simulink model "fim_15_invert"  (R2020b)
settings: Solver=ode4  StartTime=0.0  StopTime=100  RelTol=1e-3  EnableMultiTasking=on
PreLoadFcn:
  | noise_factor=1;
  | load sf_aircraft_buses;
model workspace (MAT data in the model file):
  amp_cmd = 0.119224712533
undefined symbols (not defined in the file): sf_aircraft_ModeType, sigbuilder_block
libraries: simulink x21, sf_aircraft_screen_library x7, simulink_need_slupdate x2
(part 2 of 2)

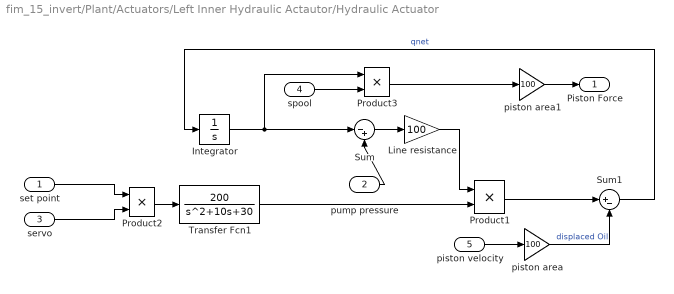
== system fim_15_invert/Plant/Actuators/Left Inner Hydraulic Actautor/Hydraulic Actuator ==
  set point : Inport
  pump pressure : Inport  Port=2
  servo : Inport  Port=3
  spool : Inport  Port=4
  piston velocity : Inport  Port=5
  Integrator : Integrator
  Line resistance : Gain  Gain=100  SaturateOnIntegerOverflow=on  OutDataTypeStr=Inherit: Same as input  ParamDataTypeStr=Inherit: Same as input
  Product1 : Product  SaturateOnIntegerOverflow=on  OutDataTypeStr=Inherit: Same as first input
  Product2 : Product  SaturateOnIntegerOverflow=on  OutDataTypeStr=Inherit: Same as first input
  Product3 : Product  SaturateOnIntegerOverflow=on  OutDataTypeStr=Inherit: Same as first input
  Sum : Sum  Inputs=|-+  SaturateOnIntegerOverflow=on
  Sum1 : Sum  Inputs=|+-  SaturateOnIntegerOverflow=on
  Transfer Fcn1 : TransferFcn  Numerator=[200]  Denominator=[1 10 30]
  piston area : Gain  Gain=100  SaturateOnIntegerOverflow=on  OutDataTypeStr=Inherit: Same as input  ParamDataTypeStr=Inherit: Same as input
  piston area1 : Gain  Gain=100  SaturateOnIntegerOverflow=on  OutDataTypeStr=Inherit: Same as input  ParamDataTypeStr=Inherit: Same as input
  Piston Force : Outport
  wires:
  spool/1 -> Product3/2
  Product3/1 -> piston area1/1
  servo/1 -> Product2/2
  Product2/1 -> Transfer Fcn1/1
  set point/1 -> Product2/1
  piston area1/1 -> Piston Force/1
  pump pressure/1 -> Sum/2
  Integrator/1 -> Sum/1, Product3/1
  Sum1/1 -> Integrator/1  "qnet"
  piston area/1 -> Sum1/2  "displaced Oil"
  piston velocity/1 -> piston area/1
  Product1/1 -> Sum1/1
  Transfer Fcn1/1 -> Product1/2
  Line resistance/1 -> Product1/1
  Sum/1 -> Line resistance/1

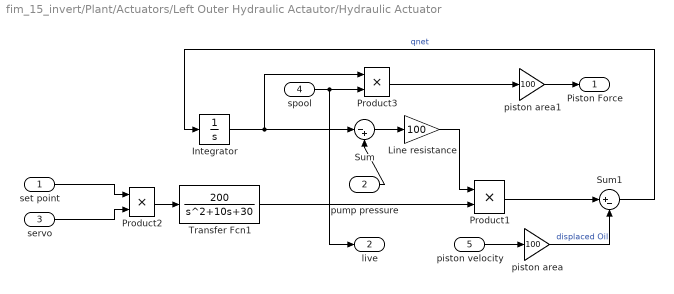
== system fim_15_invert/Plant/Actuators/Left Outer Hydraulic Actautor/Hydraulic Actuator ==
  set point : Inport
  pump pressure : Inport  Port=2
  servo : Inport  Port=3
  spool : Inport  Port=4
  piston velocity : Inport  Port=5
  Integrator : Integrator
  Line resistance : Gain  Gain=100  SaturateOnIntegerOverflow=on  OutDataTypeStr=Inherit: Same as input  ParamDataTypeStr=Inherit: Same as input
  Product1 : Product  SaturateOnIntegerOverflow=on  OutDataTypeStr=Inherit: Same as first input
  Product2 : Product  SaturateOnIntegerOverflow=on  OutDataTypeStr=Inherit: Same as first input
  Product3 : Product  SaturateOnIntegerOverflow=on  OutDataTypeStr=Inherit: Same as first input
  Sum : Sum  Inputs=|-+  SaturateOnIntegerOverflow=on
  Sum1 : Sum  Inputs=|+-  SaturateOnIntegerOverflow=on
  Transfer Fcn1 : TransferFcn  Numerator=[200]  Denominator=[1 10 30]
  piston area : Gain  Gain=100  SaturateOnIntegerOverflow=on  OutDataTypeStr=Inherit: Same as input  ParamDataTypeStr=Inherit: Same as input
  piston area1 : Gain  Gain=100  SaturateOnIntegerOverflow=on  OutDataTypeStr=Inherit: Same as input  ParamDataTypeStr=Inherit: Same as input
  Piston Force : Outport
  live : Outport  Port=2
  wires:
  spool/1 -> live/1, Product3/2
  Product3/1 -> piston area1/1
  servo/1 -> Product2/2
  Product2/1 -> Transfer Fcn1/1
  set point/1 -> Product2/1
  piston area1/1 -> Piston Force/1
  pump pressure/1 -> Sum/2
  Integrator/1 -> Sum/1, Product3/1
  Sum1/1 -> Integrator/1  "qnet"
  piston area/1 -> Sum1/2  "displaced Oil"
  piston velocity/1 -> piston area/1
  Product1/1 -> Sum1/1
  Transfer Fcn1/1 -> Product1/2
  Line resistance/1 -> Product1/1
  Sum/1 -> Line resistance/1

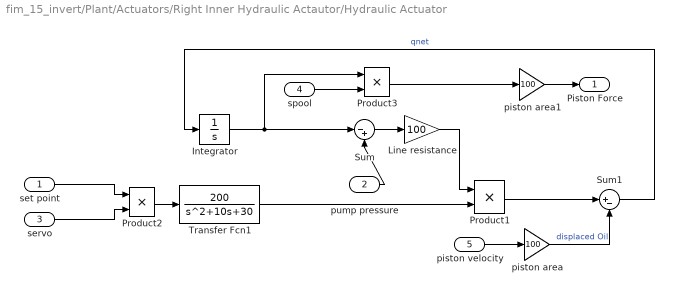
== system fim_15_invert/Plant/Actuators/Right Inner Hydraulic Actautor/Hydraulic Actuator ==
  set point : Inport
  pump pressure : Inport  Port=2
  servo : Inport  Port=3
  spool : Inport  Port=4
  piston velocity : Inport  Port=5
  Integrator : Integrator
  Line resistance : Gain  Gain=100  SaturateOnIntegerOverflow=on  OutDataTypeStr=Inherit: Same as input  ParamDataTypeStr=Inherit: Same as input
  Product1 : Product  SaturateOnIntegerOverflow=on  OutDataTypeStr=Inherit: Same as first input
  Product2 : Product  SaturateOnIntegerOverflow=on  OutDataTypeStr=Inherit: Same as first input
  Product3 : Product  SaturateOnIntegerOverflow=on  OutDataTypeStr=Inherit: Same as first input
  Sum : Sum  Inputs=|-+  SaturateOnIntegerOverflow=on
  Sum1 : Sum  Inputs=|+-  SaturateOnIntegerOverflow=on
  Transfer Fcn1 : TransferFcn  Numerator=[200]  Denominator=[1 10 30]
  piston area : Gain  Gain=100  SaturateOnIntegerOverflow=on  OutDataTypeStr=Inherit: Same as input  ParamDataTypeStr=Inherit: Same as input
  piston area1 : Gain  Gain=100  SaturateOnIntegerOverflow=on  OutDataTypeStr=Inherit: Same as input  ParamDataTypeStr=Inherit: Same as input
  Piston Force : Outport
  wires:
  spool/1 -> Product3/2
  Product3/1 -> piston area1/1
  servo/1 -> Product2/2
  Product2/1 -> Transfer Fcn1/1
  set point/1 -> Product2/1
  piston area1/1 -> Piston Force/1
  pump pressure/1 -> Sum/2
  Integrator/1 -> Sum/1, Product3/1
  Sum1/1 -> Integrator/1  "qnet"
  piston area/1 -> Sum1/2  "displaced Oil"
  piston velocity/1 -> piston area/1
  Product1/1 -> Sum1/1
  Transfer Fcn1/1 -> Product1/2
  Line resistance/1 -> Product1/1
  Sum/1 -> Line resistance/1

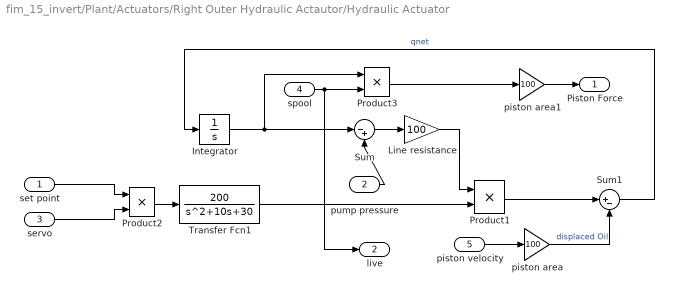
== system fim_15_invert/Plant/Actuators/Right Outer Hydraulic Actautor/Hydraulic Actuator ==
  set point : Inport
  pump pressure : Inport  Port=2
  servo : Inport  Port=3
  spool : Inport  Port=4
  piston velocity : Inport  Port=5
  Integrator : Integrator
  Line resistance : Gain  Gain=100  SaturateOnIntegerOverflow=on  OutDataTypeStr=Inherit: Same as input  ParamDataTypeStr=Inherit: Same as input
  Product1 : Product  SaturateOnIntegerOverflow=on  OutDataTypeStr=Inherit: Same as first input
  Product2 : Product  SaturateOnIntegerOverflow=on  OutDataTypeStr=Inherit: Same as first input
  Product3 : Product  SaturateOnIntegerOverflow=on  OutDataTypeStr=Inherit: Same as first input
  Sum : Sum  Inputs=|-+  SaturateOnIntegerOverflow=on
  Sum1 : Sum  Inputs=|+-  SaturateOnIntegerOverflow=on
  Transfer Fcn1 : TransferFcn  Numerator=[200]  Denominator=[1 10 30]
  piston area : Gain  Gain=100  SaturateOnIntegerOverflow=on  OutDataTypeStr=Inherit: Same as input  ParamDataTypeStr=Inherit: Same as input
  piston area1 : Gain  Gain=100  SaturateOnIntegerOverflow=on  OutDataTypeStr=Inherit: Same as input  ParamDataTypeStr=Inherit: Same as input
  Piston Force : Outport
  live : Outport  Port=2
  wires:
  spool/1 -> live/1, Product3/2
  Product3/1 -> piston area1/1
  servo/1 -> Product2/2
  Product2/1 -> Transfer Fcn1/1
  set point/1 -> Product2/1
  piston area1/1 -> Piston Force/1
  pump pressure/1 -> Sum/2
  Integrator/1 -> Sum/1, Product3/1
  Sum1/1 -> Integrator/1  "qnet"
  piston area/1 -> Sum1/2  "displaced Oil"
  piston velocity/1 -> piston area/1
  Product1/1 -> Sum1/1
  Transfer Fcn1/1 -> Product1/2
  Line resistance/1 -> Product1/1
  Sum/1 -> Line resistance/1

== system fim_15_invert/Signal conditioning and failures /Actuator Positions/Event Logging/Log LI Actuator Position Sensors ==
  In1 : Inport
  Enable : EnablePort  PropagateVarSize=During execution
  To Workspace : ToWorkspace  VariableName=LI_log  SaveFormat=Structure With Time  SampleTime=-1
  wires:
  In1/1 -> To Workspace/1  "LI_log"

== system fim_15_invert/Signal conditioning and failures /Actuator Positions/Event Logging/Log LO Actuator Position Sensors ==
  In1 : Inport
  Enable : EnablePort  PropagateVarSize=During execution
  To Workspace : ToWorkspace  VariableName=LO_log  SaveFormat=Structure With Time  SampleTime=-1
  wires:
  In1/1 -> To Workspace/1  "LO_log"

== system fim_15_invert/Signal conditioning and failures /Actuator Positions/Event Logging/Log RI Actuator Position Sensors ==
  In1 : Inport
  Enable : EnablePort  PropagateVarSize=During execution
  To Workspace : ToWorkspace  VariableName=RI_log  SaveFormat=Structure With Time  SampleTime=-1
  wires:
  In1/1 -> To Workspace/1  "RO_log"

== system fim_15_invert/Signal conditioning and failures /Actuator Positions/Event Logging/Log RO Actuator Position Sensors ==
  In1 : Inport
  Enable : EnablePort  PropagateVarSize=During execution
  To Workspace : ToWorkspace  VariableName=RO_log  SaveFormat=Structure With Time  SampleTime=-1
  wires:
  In1/1 -> To Workspace/1  "RI_log"

== system fim_15_invert/Signal conditioning and failures /Hydraulic Pressures/Event Logging/Log Hydraulic System 1 Sensors ==
  In1 : Inport
  Enable : EnablePort  PropagateVarSize=During execution
  To Workspace : ToWorkspace  VariableName=H1_log  SaveFormat=Structure With Time  SampleTime=-1
  wires:
  In1/1 -> To Workspace/1

== system fim_15_invert/Signal conditioning and failures /Hydraulic Pressures/Event Logging/Log Hydraulic System 2 Sensors ==
  In1 : Inport
  Enable : EnablePort  PropagateVarSize=During execution
  To Workspace : ToWorkspace  VariableName=H2_log  SaveFormat=Structure With Time  SampleTime=-1
  wires:
  In1/1 -> To Workspace/1  "H2_log"

== system fim_15_invert/Signal conditioning and failures /Hydraulic Pressures/Event Logging/Log Hydraulic System 3 Sensors ==
  In1 : Inport
  Enable : EnablePort  PropagateVarSize=During execution
  To Workspace : ToWorkspace  VariableName=H3_log  SaveFormat=Structure With Time  SampleTime=-1
  wires:
  In1/1 -> To Workspace/1  "H3_log"

== system fim_15_invert/Signal conditioning and failures /Hydraulic Pressures/Measured Hydraulic system 1 pressures/Hydraulic pressure ==
  H1_fail : Constant  Value=0  OutDataTypeStr=boolean
  Outlier/failure : Subsystem  Tag=STV Subsys  LoadFcn=sigbuilder_block('load');  StartFcn=sigbuilder_block('start');  StopFcn=sigbuilder_block('stop');  ClipboardFcn=sigbuilder_block('clipboard');  mask(Sigbuilder block){tuvar=[0:10]}
      mask help: Sigbuilder GUI
      mask init:
      | if ~strcmp(get_param(bdroot,'SimulationStatus'),'stopped') tuvar = sigbuilder_block('maskInit'); end
      settings: CopyFcn=sigbuilder_block('copy');  DeleteFcn=sigbuilder_block('delete');  ModelCloseFcn=sigbuilder_block('modelClose');  PreSaveFcn=sigbuilder_block('preSave');  PauseFcn=sigbuilder_block('pause')  ContinueFcn=sigbuilder_block('continue')  NameChangeFcn=sigbuilder_block('namechange');  OpenFcn=sigbuilder_block('open',[81 97.5 519.75 399.75 ]);  CloseFcn=sigbuilder_block('close');
      mask Display: plot(0, 0, 100, 100,[2, 2, 32, 32, 2], [68, 8, 8, 68, 68],[32, 2], [38, 38], [32, 19, 2],[53, 60, 44], [32, 17, 17, 2],[16, 16, 31, 31]);txt = getActiveGroup(gcbh);text(2, 100, txt,'verticalAlignment', 'top');
  Pump Pressure : Constant  Value=1000
  Switch : Switch  Criteria=u2 ~= 0  SaturateOnIntegerOverflow=on
  Out1 : Outport
  wires:
  Pump Pressure/1 -> Switch/3
  Switch/1 -> Out1/1
  Outlier/failure/1(Signal 1) -> Switch/1
  H1_fail/1 -> Switch/2

== system fim_15_invert/Signal conditioning and failures /Hydraulic Pressures/Measured Hydraulic system 1 pressures/pressure reading1 ==
  pressure : Inport
  Band-Limited White Noise : simulink/Sources/Band-Limited White Noise  Cov=[0.1]*noise_factor  Ts=0.01  seed=[25341]
  Sum : Sum  Inputs=|++  SaturateOnIntegerOverflow=on
  Out1 : Outport
  wires:
  Sum/1 -> Out1/1
  pressure/1 -> Sum/1
  Band-Limited White Noise/1 -> Sum/2

== system fim_15_invert/Signal conditioning and failures /Hydraulic Pressures/Measured Hydraulic system 1 pressures/pressure reading2 ==
  pressure : Inport
  Band-Limited White Noise : simulink/Sources/Band-Limited White Noise  Cov=[0.1]*noise_factor  Ts=0.01  seed=[21311]
  Sum1 : Sum  Inputs=|++  SaturateOnIntegerOverflow=on
  Out1 : Outport
  wires:
  Band-Limited White Noise/1 -> Sum1/2
  pressure/1 -> Sum1/1
  Sum1/1 -> Out1/1

== system fim_15_invert/Signal conditioning and failures /Hydraulic Pressures/Measured Hydraulic system 1 pressures/pressure reading3 ==
  pressure : Inport
  Band-Limited White Noise : simulink/Sources/Band-Limited White Noise  Cov=[0.1]*noise_factor  Ts=0.01  seed=[341]
  Sum1 : Sum  Inputs=|++  SaturateOnIntegerOverflow=on
  Out1 : Outport
  wires:
  Sum1/1 -> Out1/1
  pressure/1 -> Sum1/1
  Band-Limited White Noise/1 -> Sum1/2

== system fim_15_invert/Signal conditioning and failures /Hydraulic Pressures/Measured Hydraulic system 2 pressures/Hydraulic pressure ==
  H2_fail : Constant  Value=0  OutDataTypeStr=boolean
  Outlier/failure : Subsystem  Tag=STV Subsys  LoadFcn=sigbuilder_block('load');  StartFcn=sigbuilder_block('start');  StopFcn=sigbuilder_block('stop');  ClipboardFcn=sigbuilder_block('clipboard');  mask(Sigbuilder block){tuvar=[0:10]}
      mask help: Sigbuilder GUI
      mask init:
      | if ~strcmp(get_param(bdroot,'SimulationStatus'),'stopped') tuvar = sigbuilder_block('maskInit'); end
      settings: CopyFcn=sigbuilder_block('copy');  DeleteFcn=sigbuilder_block('delete');  ModelCloseFcn=sigbuilder_block('modelClose');  PreSaveFcn=sigbuilder_block('preSave');  PauseFcn=sigbuilder_block('pause')  ContinueFcn=sigbuilder_block('continue')  NameChangeFcn=sigbuilder_block('namechange');  OpenFcn=sigbuilder_block('open',[81 97.5 519.75 399.75 ]);  CloseFcn=sigbuilder_block('close');
      mask Display: plot(0, 0, 100, 100,[2, 2, 32, 32, 2], [68, 8, 8, 68, 68],[32, 2], [38, 38], [32, 19, 2],[53, 60, 44], [32, 17, 17, 2],[16, 16, 31, 31]);txt = getActiveGroup(gcbh);text(2, 100, txt,'verticalAlignment', 'top');
  Pump Pressure : Constant  Value=1000
  Switch : Switch  Criteria=u2 ~= 0  SaturateOnIntegerOverflow=on
  Out1 : Outport
  wires:
  Pump Pressure/1 -> Switch/3
  Switch/1 -> Out1/1
  Outlier/failure/1(Signal 1) -> Switch/1
  H2_fail/1 -> Switch/2

== system fim_15_invert/Signal conditioning and failures /Hydraulic Pressures/Measured Hydraulic system 2 pressures/pressure reading1 ==
  pressure : Inport
  Band-Limited White Noise : simulink/Sources/Band-Limited White Noise  Cov=[0.1]*noise_factor  Ts=0.01  seed=[25341]
  Sum : Sum  Inputs=|++  SaturateOnIntegerOverflow=on
  Out1 : Outport
  wires:
  Band-Limited White Noise/1 -> Sum/2
  pressure/1 -> Sum/1
  Sum/1 -> Out1/1

== system fim_15_invert/Signal conditioning and failures /Hydraulic Pressures/Measured Hydraulic system 2 pressures/pressure reading2 ==
  pressure : Inport
  Band-Limited White Noise : simulink/Sources/Band-Limited White Noise  Cov=[0.1]*noise_factor  Ts=0.01  seed=[21311]
  Sum1 : Sum  Inputs=|++  SaturateOnIntegerOverflow=on
  Out1 : Outport
  wires:
  Sum1/1 -> Out1/1
  pressure/1 -> Sum1/1
  Band-Limited White Noise/1 -> Sum1/2

== system fim_15_invert/Signal conditioning and failures /Hydraulic Pressures/Measured Hydraulic system 2 pressures/pressure reading3 ==
  pressure : Inport
  Band-Limited White Noise : simulink/Sources/Band-Limited White Noise  Cov=[0.1]*noise_factor  Ts=0.01  seed=[341]
  Sum1 : Sum  Inputs=|++  SaturateOnIntegerOverflow=on
  Out1 : Outport
  wires:
  Band-Limited White Noise/1 -> Sum1/2
  pressure/1 -> Sum1/1
  Sum1/1 -> Out1/1

== system fim_15_invert/Signal conditioning and failures /Hydraulic Pressures/Measured Hydraulic system 3 pressures/Hydraulic pressure ==
  H3_fail : Constant  Value=0  OutDataTypeStr=boolean
  Outlier/failure : Subsystem  Tag=STV Subsys  LoadFcn=sigbuilder_block('load');  StartFcn=sigbuilder_block('start');  StopFcn=sigbuilder_block('stop');  ClipboardFcn=sigbuilder_block('clipboard');  mask(Sigbuilder block){tuvar=[0:10]}
      mask help: Sigbuilder GUI
      mask init:
      | if ~strcmp(get_param(bdroot,'SimulationStatus'),'stopped') tuvar = sigbuilder_block('maskInit'); end
      settings: CopyFcn=sigbuilder_block('copy');  DeleteFcn=sigbuilder_block('delete');  ModelCloseFcn=sigbuilder_block('modelClose');  PreSaveFcn=sigbuilder_block('preSave');  PauseFcn=sigbuilder_block('pause')  ContinueFcn=sigbuilder_block('continue')  NameChangeFcn=sigbuilder_block('namechange');  OpenFcn=sigbuilder_block('open',[81 97.5 519.75 399.75 ]);  CloseFcn=sigbuilder_block('close');
      mask Display: plot(0, 0, 100, 100,[2, 2, 32, 32, 2], [68, 8, 8, 68, 68],[32, 2], [38, 38], [32, 19, 2],[53, 60, 44], [32, 17, 17, 2],[16, 16, 31, 31]);txt = getActiveGroup(gcbh);text(2, 100, txt,'verticalAlignment', 'top');
  Pump Pressure : Constant  Value=1000
  Switch : Switch  Criteria=u2 ~= 0  SaturateOnIntegerOverflow=on
  Out1 : Outport
  wires:
  Pump Pressure/1 -> Switch/3
  Switch/1 -> Out1/1
  Outlier/failure/1(Signal 1) -> Switch/1
  H3_fail/1 -> Switch/2

== system fim_15_invert/Signal conditioning and failures /Hydraulic Pressures/Measured Hydraulic system 3 pressures/pressure reading1 ==
  pressure : Inport
  Band-Limited White Noise : simulink/Sources/Band-Limited White Noise  Cov=[0.1]*noise_factor  Ts=0.01  seed=[2341]
  Sum : Sum  Inputs=|++  SaturateOnIntegerOverflow=on
  Out1 : Outport
  wires:
  Sum/1 -> Out1/1
  pressure/1 -> Sum/1
  Band-Limited White Noise/1 -> Sum/2

== system fim_15_invert/Signal conditioning and failures /Hydraulic Pressures/Measured Hydraulic system 3 pressures/pressure reading2 ==
  pressure : Inport
  Band-Limited White Noise : simulink/Sources/Band-Limited White Noise  Cov=[0.1]*noise_factor  Ts=0.01  seed=[1311]
  Sum1 : Sum  Inputs=|++  SaturateOnIntegerOverflow=on
  Out1 : Outport
  wires:
  Band-Limited White Noise/1 -> Sum1/2
  pressure/1 -> Sum1/1
  Sum1/1 -> Out1/1

== system fim_15_invert/Signal conditioning and failures /Hydraulic Pressures/Measured Hydraulic system 3 pressures/pressure reading3 ==
  pressure : Inport
  Band-Limited White Noise : simulink/Sources/Band-Limited White Noise  Cov=[0.1]*noise_factor  Ts=0.01  seed=[1341]
  Sum1 : Sum  Inputs=|++  SaturateOnIntegerOverflow=on
  Out1 : Outport
  wires:
  Sum1/1 -> Out1/1
  pressure/1 -> Sum1/1
  Band-Limited White Noise/1 -> Sum1/2

== system fim_15_invert/Signal conditioning and failures /Hydraulic Pressures/Measured Hydraulic system 1 pressures/Hydraulic pressure/Outlier//failure ==
  Demux : Demux  Tag=STV Demux  Outputs=1
      settings: DisplayOption=none
  FromWs : FromWorkspace  Tag=STV FromWs  VariableName=tuvar  ZeroCross=off
      SigBuilderData=|
      | dataSet.timeRange = [0 30]
      | dataSet.name = 'Group 1'
      | sbobj.Groups.Name = 'Group 1'
      | sbobj.Groups.Signals.Name = 'Signal 1'
      | sbobj.Groups.Signals.XData = [0 30]
      | sbobj.Groups.Signals.YData = [100 100]
      | sbobj.Groups.TimeRange = [0 30]
  Signal 1 : Outport  Tag=STV Outport
  wires:
  FromWs/1 -> Demux/1
  Demux/1 -> Signal 1/1

== system fim_15_invert/Signal conditioning and failures /Hydraulic Pressures/Measured Hydraulic system 2 pressures/Hydraulic pressure/Outlier//failure ==
  Demux : Demux  Tag=STV Demux  Outputs=1
      settings: DisplayOption=none
  FromWs : FromWorkspace  Tag=STV FromWs  VariableName=tuvar  ZeroCross=off
      SigBuilderData=|
      | dataSet.timeRange = [0 30]
      | dataSet.name = 'Group 1'
      | sbobj.Groups.Name = 'Group 1'
      | sbobj.Groups.Signals.Name = 'Signal 1'
      | sbobj.Groups.Signals.XData = [0 30]
      | sbobj.Groups.Signals.YData = [100 100]
      | sbobj.Groups.TimeRange = [0 30]
  Signal 1 : Outport  Tag=STV Outport
  wires:
  FromWs/1 -> Demux/1
  Demux/1 -> Signal 1/1

== system fim_15_invert/Signal conditioning and failures /Hydraulic Pressures/Measured Hydraulic system 3 pressures/Hydraulic pressure/Outlier//failure ==
  Demux : Demux  Tag=STV Demux  Outputs=1
      settings: DisplayOption=none
  FromWs : FromWorkspace  Tag=STV FromWs  VariableName=tuvar  ZeroCross=off
      SigBuilderData=|
      | dataSet.timeRange = [0 30]
      | dataSet.name = 'Group 1'
      | sbobj.Groups.Name = 'Group 1'
      | sbobj.Groups.Signals.Name = 'Signal 1'
      | sbobj.Groups.Signals.XData = [0 30]
      | sbobj.Groups.Signals.YData = [100 100]
      | sbobj.Groups.TimeRange = [0 30]
  Signal 1 : Outport  Tag=STV Outport
  wires:
  FromWs/1 -> Demux/1
  Demux/1 -> Signal 1/1

== stateflow chart fim_15_invert/Mode Logic ==
  settings: sampleTime=0.5
  state Actuators
    en:L_switch();R_switch();
    du:L_switch();R_switch();
    state LO [parallel]
      settings: executionOrder=1
      state L1
        state Passive
        state Active
        state Standby
        state Off
          ex:fails++;
        (default) -> Actuators.LO.L1.Passive
        Actuators.LO.L1.Passive -> (junction 147) [order 2]
        (junction 147) -> Actuators.LO.L1.Active : [!LI_act()|RO_act()]
        Actuators.LO.L1.Active -> Actuators.LO.L1.Standby : [!RO_act()&&...
            | LI_act()]
        Actuators.LO.L1.Standby -> (junction 147)
        Actuators.LO.L1.Passive -> Actuators.LO.L1.Standby [order 1] : [LI_act()]
        Actuators.LO.L1 -> (junction 141) [order 1] : go_off[!in(Off)]
        (junction 141) -> Actuators.LO.L1.Off [order 2] : /send(E,LI);
        Actuators.LO.L1.Off -> Actuators.LO.L1 : [!u.low_press[0]]
      state Isolated
      (default) -> Actuators.LO.L1
      (junction 141) -> Actuators.LO.Isolated [order 1] : [fails>=5]
      Actuators.LO.L1 -> Actuators.LO.Isolated [order 1] : go_isolated/...
          | send(E,LI);
    state RO [parallel]
      settings: executionOrder=2
      state L1
        state Passive
        state Active
        state Standby
        state Off
          ex:fails++;
        (default) -> Actuators.RO.L1.Passive
        Actuators.RO.L1.Passive -> (junction 154) [order 2]
        (junction 154) -> Actuators.RO.L1.Active : [!RI_act()|LO_act()]
        Actuators.RO.L1.Standby -> (junction 154)
        Actuators.RO.L1.Active -> Actuators.RO.L1.Standby : [!LO_act()&&...
            | RI_act()]
        Actuators.RO.L1.Passive -> Actuators.RO.L1.Standby [order 1] : [RI_act()]
        Actuators.RO.L1.Off -> Actuators.RO.L1 : [!u.low_press[2]]
        Actuators.RO.L1 -> (junction 153) [order 1] : go_off[!in(Off)]
        (junction 153) -> Actuators.RO.L1.Off [order 2] : /send(E,RI);
      state Isolated
      (default) -> Actuators.RO.L1
      (junction 153) -> Actuators.RO.Isolated [order 1] : [fails>=5]
      Actuators.RO.L1 -> Actuators.RO.Isolated [order 1] : go_isolated/send(E,RI);
    state LI [parallel]
      settings: executionOrder=3
      state L1
        state Passive
        state Active
          entry: send(E,LO);
        state Standby
        state Off
          ex:fails++;
        (default) -> Actuators.LI.L1.Passive
        Actuators.LI.L1.Passive -> (junction 152) [order 2]
        (junction 152) -> Actuators.LI.L1.Active : [!LO_act()|RI_act()]
        Actuators.LI.L1.Standby -> (junction 152)
        Actuators.LI.L1.Passive -> Actuators.LI.L1.Standby [order 1] : [LO_act()]
        Actuators.LI.L1.Active -> Actuators.LI.L1.Standby : [RO_act()&&...
            | LO_act()]
        Actuators.LI.L1.Off -> Actuators.LI.L1 : [!u.low_press[1]]
        Actuators.LI.L1 -> (junction 151) [order 1] : go_off[!in(Off)]
        (junction 151) -> Actuators.LI.L1.Off [order 2] : /send(E,LO);...
            | send(E,RO);
      state Isolated
      (default) -> Actuators.LI.L1
      (junction 151) -> Actuators.LI.Isolated [order 1] : [fails>=5]
      Actuators.LI.L1 -> Actuators.LI.Isolated [order 1] : go_isolated/send(E,LO);...
          | send(E,RO);
    state RI [parallel]
      settings: executionOrder=4
      state L1
        state Passive
        state Active
          entry: send(E,RO);
        state Standby
        state Off
          ex:fails++;
        (default) -> Actuators.RI.L1.Passive
        Actuators.RI.L1.Passive -> (junction 150) [order 2]
        (junction 150) -> Actuators.RI.L1.Active : [!RO_act()|LI_act()]
        Actuators.RI.L1.Standby -> (junction 150)
        Actuators.RI.L1.Passive -> Actuators.RI.L1.Standby [order 1] : [RO_act()]
        Actuators.RI.L1.Active -> Actuators.RI.L1.Standby : [LO_act()&&...
            | RO_act()]
        Actuators.RI.L1 -> (junction 149) [order 1] : go_off[!in(Off)]
        (junction 149) -> Actuators.RI.L1.Off [order 2] : /send(E,RO);...
            | send(E,LO);send(E,LI);
        Actuators.RI.L1.Off -> Actuators.RI.L1 : [!u.low_press[1]]
      state Isolated
      (default) -> Actuators.RI.L1
      (junction 149) -> Actuators.RI.Isolated [order 1] : [fails>=5]
      Actuators.RI.L1 -> Actuators.RI.Isolated [order 1] : go_isolated/send(E,RO);...
          | send(E,LO);send(E,LI);
  state L_switch [function]
    (default) -> (junction 810)
    (junction 810) -> (junction 812) : {
        | /* Hydraulic system 1 Low pressure (Left Outer line) */
        | aVarTruthTableCondition_1 = (u.low_press[0]);
        | }
    (junction 812) -> (junction 814) : {
        | /* Left Outer actuator position failed */
        | aVarTruthTableCondition_2 = (u.L_pos_fail[0]);
        | }
    (junction 814) -> (junction 816) : {
        | /* Hydraulic system 2 Low pressure (Inner line) */
        | aVarTruthTableCondition_3 = (u.low_press[1]);
        | }
    (junction 816) -> (junction 818) : {
        | /* Left Inner actuator position failed */
        | aVarTruthTableCondition_4 = (u.L_pos_fail[1]);
        | }
    (junction 818) -> (junction 820) [order 1] : [aVarTruthTableCondition_1 && !aVarTruthTableCondition_3 && !aVarTruthTableCondition_4]
    (junction 820) -> (junction 822) : {
        | /* Hydraulic System 1 Failure. Turn off Left Outer Actuator */
        | send(go_off,Actuators.LO);
        | }
    (junction 818) -> (junction 824) [order 2]
    (junction 824) -> (junction 826) [order 1] : [aVarTruthTableCondition_1]
    (junction 826) -> (junction 828) : {
        | /* Left Outer Actuator Failure. Isolate Left Outer Actuator */
        | send(go_isolated,Actuators.LO);
        | }
    (junction 828) -> (junction 830) : {
        | /* Left Inner Actuator Failure. Isolate Left Inner Actuator */
        | send(go_isolated,Actuators.LI);
        | }
    (junction 824) -> (junction 832) [order 2]
    (junction 832) -> (junction 834) [order 1] : [!aVarTruthTableCondition_1 && aVarTruthTableCondition_2 && !aVarTruthTableCondition_3 && !aVarTruthTableCondition_4]
    (junction 834) -> (junction 836) : {
        | /* Left Outer Actuator Failure. Isolate Left Outer Actuator */
        | send(go_isolated,Actuators.LO);
        | }
    (junction 832) -> (junction 838) [order 2]
    (junction 838) -> (junction 840) [order 1] : [!aVarTruthTableCondition_1 && aVarTruthTableCondition_2]
    (junction 840) -> (junction 842) : {
        | /* Left Outer Actuator Failure. Isolate Left Outer Actuator */
        | send(go_isolated,Actuators.LO);
        | }
    (junction 842) -> (junction 844) : {
        | /* Left Inner Actuator Failure. Isolate Left Inner Actuator */
        | send(go_isolated,Actuators.LI);
        | }
    (junction 838) -> (junction 846) [order 2]
    (junction 846) -> (junction 848) [order 1] : [aVarTruthTableCondition_3]
    (junction 848) -> (junction 850) : {
        | /* Hydraulic System 2 Failure. Turn off Left Inner Actuator */
        | send(go_off,Actuators.LI);
        | }
    (junction 846) -> (junction 852) [order 2]
    (junction 852) -> (junction 854) [order 1] : [aVarTruthTableCondition_4]
    (junction 854) -> (junction 856) : {
        | /* Left Inner Actuator Failure. Isolate Left Inner Actuator */
        | send(go_isolated,Actuators.LI);
        | }
    (junction 852) -> (junction 858) [order 2]
    (junction 858) -> (junction 860) : /* Default */
    (junction 860) -> (junction 862) : {
        | /* 'Default':Default - All ok, do nothing. */
        |
        | }
  state R_switch [function]
    (default) -> (junction 927)
    (junction 927) -> (junction 929) : {
        | /* Hydraulic system 3 Low pressure (Right Outer line) */
        | aVarTruthTableCondition_1 = (u.low_press[2]);
        | }
    (junction 929) -> (junction 931) : {
        | /* Right Outer actuator position failed */
        | aVarTruthTableCondition_2 = (u.R_pos_fail[0]);
        | }
    (junction 931) -> (junction 933) : {
        | /* Hydraulic system 2 Low pressure (Inner line) */
        | aVarTruthTableCondition_3 = (u.low_press[1]);
        | }
    (junction 933) -> (junction 935) : {
        | /* Right Inner actuator position failed */
        | aVarTruthTableCondition_4 = (u.R_pos_fail[1]);
        | }
    (junction 935) -> (junction 937) [order 1] : [aVarTruthTableCondition_1 && !aVarTruthTableCondition_3 && !aVarTruthTableCondition_4]
    (junction 937) -> (junction 939) : {
        | /* Hydraulic System 3 Failure. Turn off Right Outer Actuator */
        | send(go_off,Actuators.RO);
        | }
    (junction 935) -> (junction 941) [order 2]
    (junction 941) -> (junction 943) [order 1] : [aVarTruthTableCondition_1]
    (junction 943) -> (junction 945) : {
        | /* Multiple Failure. Isolate Right Outer AND Right Inner Actuators */
        | send(go_isolated,Actuators.RO);
        | send(go_isolated,Actuators.RI);
        | }
    (junction 941) -> (junction 947) [order 2]
    (junction 947) -> (junction 949) [order 1] : [!aVarTruthTableCondition_1 && aVarTruthTableCondition_2 && !aVarTruthTableCondition_3 && !aVarTruthTableCondition_4]
    (junction 949) -> (junction 951) : {
        | /* Right Outer Actuator Failure. Isolate Right Outer Actuator */
        | send(go_isolated,Actuators.RO);
        | }
    (junction 947) -> (junction 953) [order 2]
    (junction 953) -> (junction 955) [order 1] : [!aVarTruthTableCondition_1 && aVarTruthTableCondition_2]
    (junction 955) -> (junction 957) : {
        | /* Multiple Failure. Isolate Right Outer AND Right Inner Actuators */
        | send(go_isolated,Actuators.RO);
        | send(go_isolated,Actuators.RI);
        | }
    (junction 953) -> (junction 959) [order 2]
    (junction 959) -> (junction 961) [order 1] : [aVarTruthTableCondition_3]
    (junction 961) -> (junction 963) : {
        | /* Hydraulic System 2 Failure. Turn off Right Inner Actuator */
        | send(go_off,Actuators.RI);
        | }
    (junction 959) -> (junction 965) [order 2]
    (junction 965) -> (junction 967) [order 1] : [aVarTruthTableCondition_4]
    (junction 967) -> (junction 969) : {
        | /* Right Inner Actuator Failure. Isolate Right Inner Actuator */
        | send(go_isolated,Actuators.RI);
        | }
    (junction 965) -> (junction 971) [order 2]
    (junction 971) -> (junction 973) : /* Default */
    (junction 973) -> (junction 975) : {
        | /* 'Default':Default - All ok, do nothing. */
        |
        | }
  state y_act = LO_act [function]
    (default) -> (junction 159) : {y_act=in(Actuators.LO.L1.Active);}
  state y_act = LI_act [function]
    (default) -> (junction 160) : {y_act=in(Actuators.LI.L1.Active);}
  state y_act = RO_act [function]
    (default) -> (junction 158) : {y_act=in(Actuators.RO.L1.Active);}
  state y_act = RI_act [function]
    (default) -> (junction 157) : {y_act=in(Actuators.RI.L1.Active);}
  note: This mode logic assumes that there are 3 hydraulic lines, one that is connected to the 2 redundant actuators (Left Inner and Right Inner actuators).
      | The other two are connected to the primary actuators Left Outer and Right Outer (1 per actuator).
  data: fails local int32; fails local int32; fails local int32; fails local int32; aVarTruthTableCondition_1 temporary boolean =0; aVarTruthTableCondition_2 temporary boolean =0; aVarTruthTableCondition_3 temporary boolean =0; aVarTruthTableCondition_4 temporary boolean =0; aVarTruthTableCondition_1 temporary boolean =0; aVarTruthTableCondition_2 temporary boolean =0; aVarTruthTableCondition_3 temporary boolean =0; aVarTruthTableCondition_4 temporary boolean =0; y_act function_output double; y_act function_output double; y_act function_output double; y_act function_output double; u input Bus: PositionBus size=1; LO_mode output Enum: sf_aircraft_ModeType; RO_mode output Enum: sf_aircraft_ModeType; LI_mode output Enum: sf_aircraft_ModeType; RI_mode output Enum: sf_aircraft_ModeType
  data aVarTruthTableCondition_1 settings: description=Hydraulic system 1 Low pressure (Left Outer line)
  data aVarTruthTableCondition_2 settings: description=Left Outer actuator position failed
  data aVarTruthTableCondition_3 settings: description=Hydraulic system 2 Low pressure (Inner line)
  data aVarTruthTableCondition_4 settings: description=Left Inner actuator position failed
  data aVarTruthTableCondition_1 settings: description=Hydraulic system 3 Low pressure (Right Outer line)
  data aVarTruthTableCondition_2 settings: description=Right Outer actuator position failed
  data aVarTruthTableCondition_3 settings: description=Hydraulic system 2 Low pressure (Inner line)
  data aVarTruthTableCondition_4 settings: description=Right Inner actuator position failed
  events: go_isolated local EITHER_EDGE_EVENT; go_off local EITHER_EDGE_EVENT; E local EITHER_EDGE_EVENT
